simulink model "W2Q4"  (R2020a)
settings: Solver=VariableStepAuto  StartTime=0.0  StopTime=10.0  RelTol=1e-3
values from neighbouring files (symbols this model uses):
  b = 3.5077*(10^(-6))    (= 3.5077e-06)    [para.m]
  J = 3.228*(10^(-6))    (= 3.228e-06)    [para.m]
  ke = 0.0274    [para.m]
  kt = 0.0274    [para.m]
  L = 2.75*(10^(-6))    (= 2.75e-06)    [para.m]
  R = 4    [para.m]
settings Model: Creator=Vinayak  LastModifiedBy=Vinayak

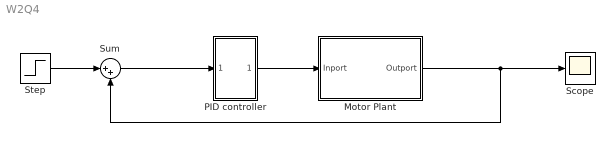
== system W2Q4 ==
  Motor Plant : Subsystem
  PID controller : Subsystem
  Scope : Scope
  Step : Step  Time=0  SampleTime=0
  Sum : Sum  Inputs=|++
  wires:
  Step/1 -> Sum/1
  Motor Plant/1(Outport) -> Scope/1, Sum/2
  Sum/1 -> PID controller/1(In1)
  PID controller/1(Inport) -> Motor Plant/1(Inport)

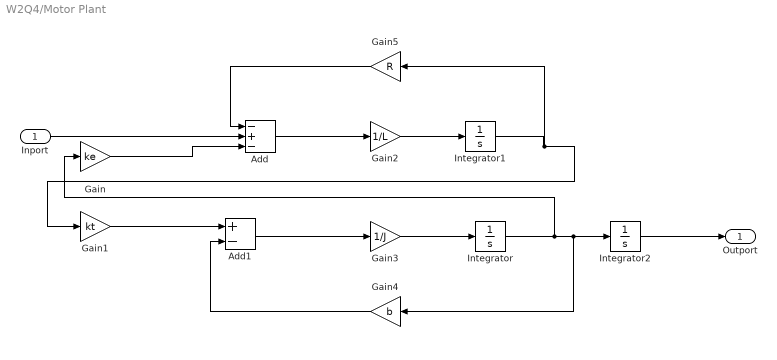
== system W2Q4/Motor Plant ==
  Inport : Inport
  Add : Sum  Inputs=-+-
  Add1 : Sum  Inputs=+-
  Gain : Gain  Gain=ke
  Gain1 : Gain  Gain=kt
  Gain2 : Gain  Gain=1/L
  Gain3 : Gain  Gain=1/J
  Gain4 : Gain  Gain=b
  Gain5 : Gain  Gain=R
  Integrator : Integrator
  Integrator1 : Integrator
  Integrator2 : Integrator
  Outport : Outport
  wires:
  Add1/1 -> Gain3/1
  Inport/1 -> Add/2
  Gain/1 -> Add/3
  Gain1/1 -> Add1/1
  Gain4/1 -> Add1/2
  Gain5/1 -> Add/1
  Gain2/1 -> Integrator1/1
  Integrator/1 -> Integrator2/1, Gain4/1, Gain/1
  Add/1 -> Gain2/1
  Integrator1/1 -> Gain5/1, Gain1/1
  Integrator2/1 -> Outport/1
  Gain3/1 -> Integrator/1

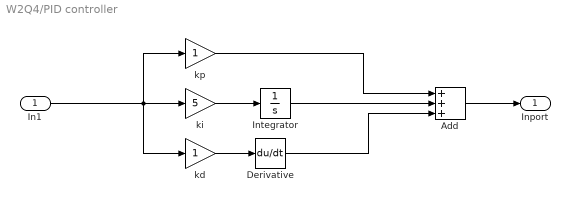
== system W2Q4/PID controller ==
  In1 : Inport
  Add : Sum  Inputs=+++
  Derivative : Derivative
  Integrator : Integrator
  kd : Gain
  ki : Gain  Gain=5
  kp : Gain
  Inport : Outport
  wires:
  Add/1 -> Inport/1
  kd/1 -> Derivative/1
  ki/1 -> Integrator/1
  Integrator/1 -> Add/2
  Derivative/1 -> Add/3
  kp/1 -> Add/1
  In1/1 -> kd/1, ki/1, kp/1
